simulink model "mStateflow"  (R2021b)
settings: Solver=VariableStepAuto  StartTime=0.0  StopTime=10.0  RelTol=1e-3
settings Model: Creator=anitschk  LastModifiedBy=anitschk

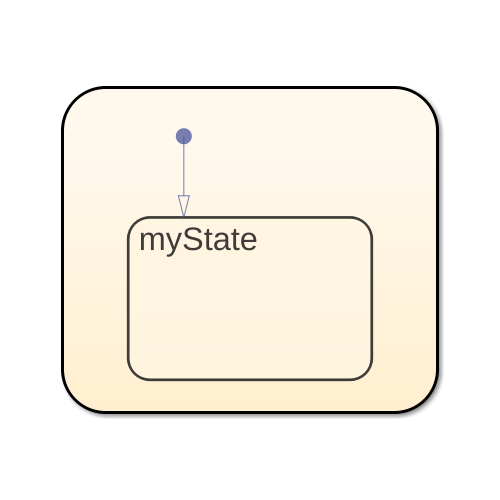
[thumbnail: Simulink's stored preview of the top-level diagram]
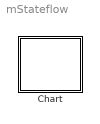
== system mStateflow ==
  Chart : Stateflow chart  TreatAsAtomicUnit=on

== stateflow chart mStateflow/Chart ==
  state myState
  (default) -> myState
